simulink model "Drv002"  (Simulink 8.3)
settings: Solver=ode45  StartTime=0.0  StopTime=10.0  RelTol=1e-3
model workspace (MAT data in the model file):
  pDrv : struct (value not decoded)
settings Model: Creator=swami  LastModifiedBy=swami
settings DataIOCC: SignalLoggingSaveFormat=Dataset
settings DebuggingCC: UnderspecifiedInitializationDetection=Simplified  StateNameClashWarn=none
settings GRTTargetCC: CombineOutputUpdateFcns=on  GRTInterface=off

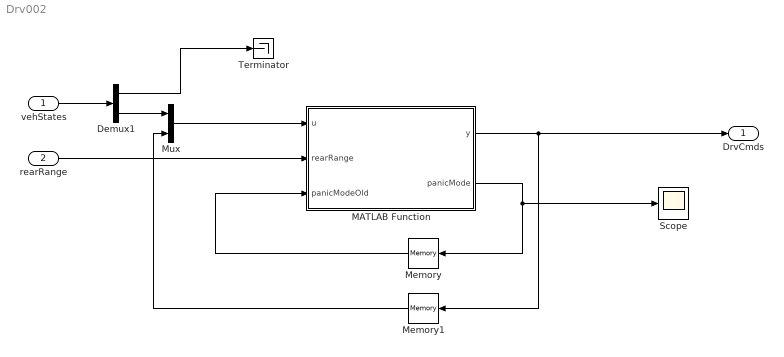
== system Drv002 ==
  vehStates : Inport
  rearRange : Inport  Port=2
  Demux1 : Demux  Outputs=2
  MATLAB Function : MATLAB Function  TreatAsAtomicUnit=on
  Memory : Memory
  Memory1 : Memory  X0=[0,0,0,0]
  Mux : Mux  Inputs=2
  Scope : Scope
  Terminator : Terminator
  DrvCmds : Outport
  wires:
  MATLAB Function/1(y) -> Memory1/1, DrvCmds/1
  vehStates/1 -> Demux1/1
  Demux1/1 -> Terminator/1
  Demux1/2 -> Mux/1
  Mux/1 -> MATLAB Function/1(u)
  Memory1/1 -> Mux/2
  rearRange/1 -> MATLAB Function/2(rearRange)
  MATLAB Function/2(panicMode) -> Scope/1, Memory/1
  Memory/1 -> MATLAB Function/3(panicModeOld)

== matlab function MATLAB Function ==
  data: u input double; rearRange input double; panicModeOld input double; y output double; pDrv parameter double; panicMode output double
function [y,panicMode] = fcn(u,rearRange,panicModeOld,pDrv)
y = [0,0,0,0];
spd = u(1);
CCSw = u(4);
%CCSw = 0;

if (panicModeOld == 1)
    if (rearRange > 50.5)
        panicMode = 0;
    else
        panicMode = 1;
    end
else
    if (rearRange < 50)
        panicMode = 1;
    else
        panicMode = 0;
    end
end    


if (panicMode == 1)
    brk = 0.0;
    thr = 0.5;
    CCSw_new = 0.0;
    CCSetPt = 0.0;
else
    if (spd< pDrv.CCSetPt && CCSw<0.5)
        brk = 0.0;
        thr = 1.0;
        CCSw_new = 0.0;
        CCSetPt = 0.0;
    else
        brk = 0.0;
        thr = 0.0;
        CCSw_new = 1.0;
        CCSetPt = pDrv.CCSetPt;
    end
end


y(1) = brk;
y(2) = thr;
y(3) = CCSw_new;
y(4) = CCSetPt;
